simulink model "poleplacement"  (R2023b)
settings: Solver=VariableStepAuto  StartTime=0.0  StopTime=10.0  RelTol=1e-3
values from neighbouring files (symbols this model uses):
  A = sys_d.A    [error_dynamic.m]
  B = sys_d.B    [error_dynamic.m]
  C = sys_d.C    [error_dynamic.m]
  E = Es * Wr    [error_dynamic.m]
  K = place(A,B,p0)    [error_dynamic.m]
  Ts = 0.25    [error_dynamic.m]
  x0 = [0.8;0.2;-0.6;0]    [error_dynamic.m]
settings Model: Creator=Fan Xiuqi  LastModifiedBy=Fan Xiuqi

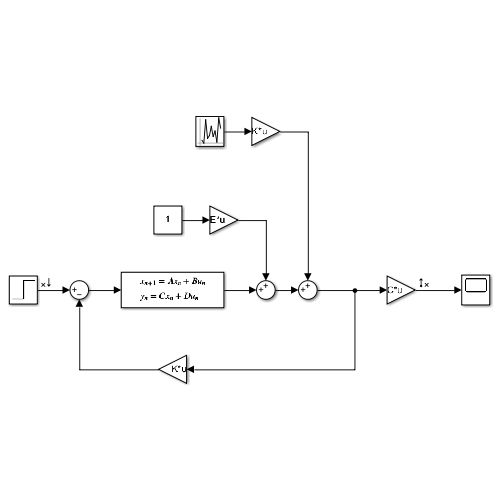
[thumbnail: Simulink's stored preview of the top-level diagram]
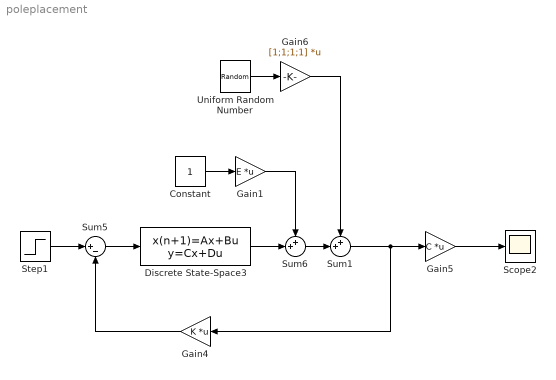
== system poleplacement ==
  Constant : Constant  SampleTime=Ts
  Discrete State-Space3 : DiscreteStateSpace  A=A  B=B  C=eye(4)  D=zeros(4,1)  InitialCondition=x0  SampleTime=Ts
  Gain1 : Gain  Gain=E  Multiplication=Matrix(K*u)
  Gain4 : Gain  Gain=K  Multiplication=Matrix(K*u)
  Gain5 : Gain  Gain=C  Multiplication=Matrix(K*u)
  Gain6 : Gain  Gain=[1;1;1;1]  Multiplication=Matrix(K*u)
  Scope2 : Scope
  Step1 : Step  SampleTime=Ts
  Sum1 : Sum  Inputs=++|
  Sum5 : Sum  Inputs=|+-
  Sum6 : Sum  Inputs=++|
  Uniform Random Number : UniformRandomNumber  Minimum=-0.2  Maximum=0.2  SampleTime=Ts
  wires:
  Step1/1 -> Sum5/1
  Discrete State-Space3/1 -> Sum6/2
  Gain5/1 -> Scope2/1
  Gain4/1 -> Sum5/2
  Sum5/1 -> Discrete State-Space3/1
  Sum6/1 -> Sum1/2
  Constant/1 -> Gain1/1
  Gain1/1 -> Sum6/1
  Sum1/1 -> Gain4/1, Gain5/1
  Uniform Random Number/1 -> Gain6/1
  Gain6/1 -> Sum1/1
